simulink library "Cloudage"  (Simulink 8.2)
settings: Solver=ode45  StartTime=0.0  StopTime=10.0  RelTol=1e-3
settings Model: Creator=drhf  LastModifiedBy=drhf

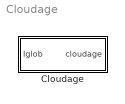
== system Cloudage ==
  Cloudage : Subsystem  mask(cloud index){latitude=51, longitude=-7, longitude0=-30, skytype=high mountain}
      mask prompts: latitude "Latitude [-90;90], north positive"; longitude "Longitude  [-180;180], west positive"; longitude0 "reference longitude (timezone)"; skytype "Sky Type"
      mask help:
      | Calculates the cloud index. The cloud index is the fraction of the sky covered by clouds in [0, 1/8, 2/8, 3/8, ..., 7/8, 1].
      |
      | INPUT VECTOR:
      |  time    : real time or simulation time [s]
      |  Iglob   : global radiation on horizontal surface (W/m²)
      |
      | OUTPUT VECTOR:
      |  cloud  : cloudindex [0;1]
      mask Help: web(fullfile(path_carnot('help'),'Cloudage.html'),'-helpbrowser')
      mask TypeOptions skytype: high mountain | lowland | urban region | industrial zone

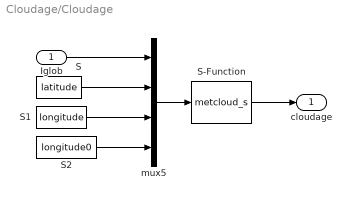
== system Cloudage/Cloudage ==
  Iglob : Inport
  S : Constant  Value=latitude
  S-Function : S-Function  FunctionName=metcloud_s  Parameters=skytype  EnableBusSupport=off
  S1 : Constant  Value=longitude
  S2 : Constant  Value=longitude0
  mux5 : Mux
  cloudage : Outport
  wires:
  Iglob/1 -> mux5/1
  S-Function/1 -> cloudage/1
  S2/1 -> mux5/4
  mux5/1 -> S-Function/1
  S/1 -> mux5/2
  S1/1 -> mux5/3
